simulink model "zad1"  (R2023b)
settings: Solver=VariableStepAuto  StartTime=0.0  StopTime=10.0  RelTol=1e-3
undefined symbols (not defined in the file): A, Ad, B, Bd, C, Cd, D, Dd, h
settings Model: Creator=roman  LastModifiedBy=roman

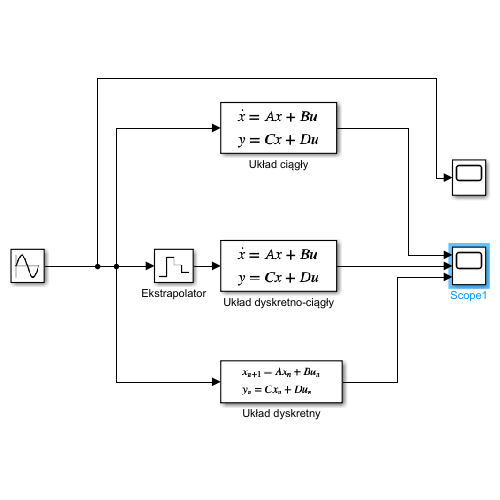
[thumbnail: Simulink's stored preview of the top-level diagram]
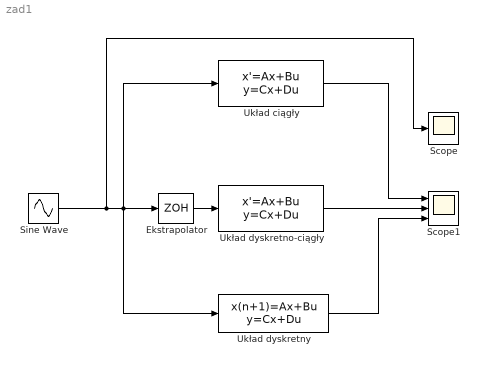
== system zad1 ==
  Ekstrapolator : ZeroOrderHold  SampleTime=h
  Scope : Scope
  Scope1 : Scope  NumInputPorts=3
  Sine Wave : Sin  SampleTime=0
  Układ ciągły : StateSpace  A=A  B=B  C=C  InitialCondition=[1 0]
  Układ dyskretno-ciągły : StateSpace  A=A  B=B  C=C  D=D  InitialCondition=[1 0]  ParameterTunability=Unconstrained
  Układ dyskretny : DiscreteStateSpace  A=Ad  B=Bd  C=Cd  D=Dd  InitialCondition=[1 0]  SampleTime=h
  wires:
  Ekstrapolator/1 -> Układ dyskretno-ciągły/1
  Sine Wave/1 -> Scope/1, Układ dyskretny/1, Układ ciągły/1, Ekstrapolator/1
  Układ ciągły/1 -> Scope1/1
  Układ dyskretno-ciągły/1 -> Scope1/2
  Układ dyskretny/1 -> Scope1/3
